simulink model "desired_dynamics"  (R2018b)
settings: Solver=ode8  StartTime=0.0  StopTime=10.0  FixedStep=0.01  RelTol=1e-3
settings Model: Creator=suvo.ganguli  LastModifiedBy=suvo.ganguli

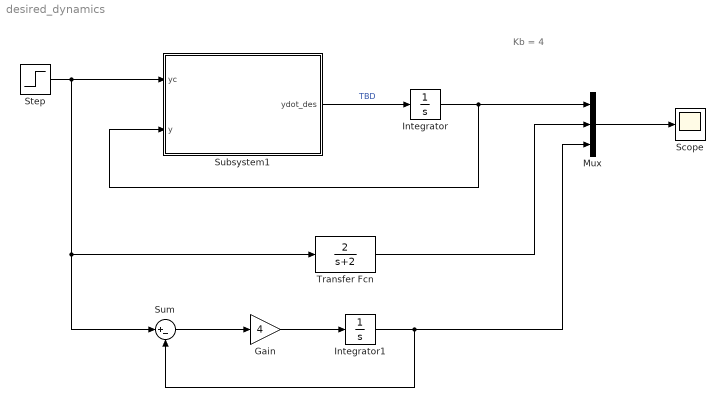
== system desired_dynamics ==
  note: Kb = 4
  Gain : Gain  Gain=4
  Integrator : Integrator
  Integrator1 : Integrator
  Mux : Mux  Inputs=3
  Scope : Scope
  Step : Step  SampleTime=0
  Subsystem1 : Subsystem
  Sum : Sum  Inputs=|+-
  Transfer Fcn : TransferFcn  Numerator=[2]  Denominator=[1 2]
  wires:
  Subsystem1/1(ydot_des) -> Integrator/1  "TBD"
  Integrator/1 -> Subsystem1/2(y), Mux/1
  Mux/1 -> Scope/1
  Step/1 -> Sum/1, Transfer Fcn/1, Subsystem1/1(yc)
  Transfer Fcn/1 -> Mux/2
  Gain/1 -> Integrator1/1
  Sum/1 -> Gain/1
  Integrator1/1 -> Mux/3, Sum/2

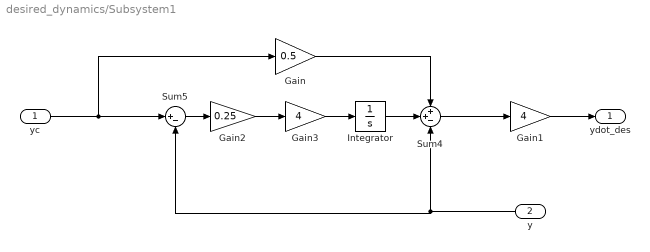
== system desired_dynamics/Subsystem1 ==
  yc : Inport
  y : Inport  Port=2
  Gain : Gain  Gain=0.5
  Gain1 : Gain  Gain=4
  Gain2 : Gain  Gain=0.25
  Gain3 : Gain  Gain=4
  Integrator : Integrator
  Sum4 : Sum  Inputs=++-
  Sum5 : Sum  Inputs=|+-
  ydot_des : Outport
  wires:
  Gain3/1 -> Integrator/1
  Sum4/1 -> Gain1/1
  Gain2/1 -> Gain3/1
  Sum5/1 -> Gain2/1
  yc/1 -> Gain/1, Sum5/1
  Integrator/1 -> Sum4/2
  Gain/1 -> Sum4/1
  y/1 -> Sum5/2, Sum4/3
  Gain1/1 -> ydot_des/1
